simulink model "Block_diagram"  (R2018b)
settings: Solver=VariableStepAuto  StartTime=0.0  StopTime=10  FixedStep=1e-6  RelTol=1e-3
undefined symbols (not defined in the file): sigbuilder_block
libraries: simulink x2
settings Model: Creator=Anmol Kathail  LastModifiedBy=Anmol Kathail

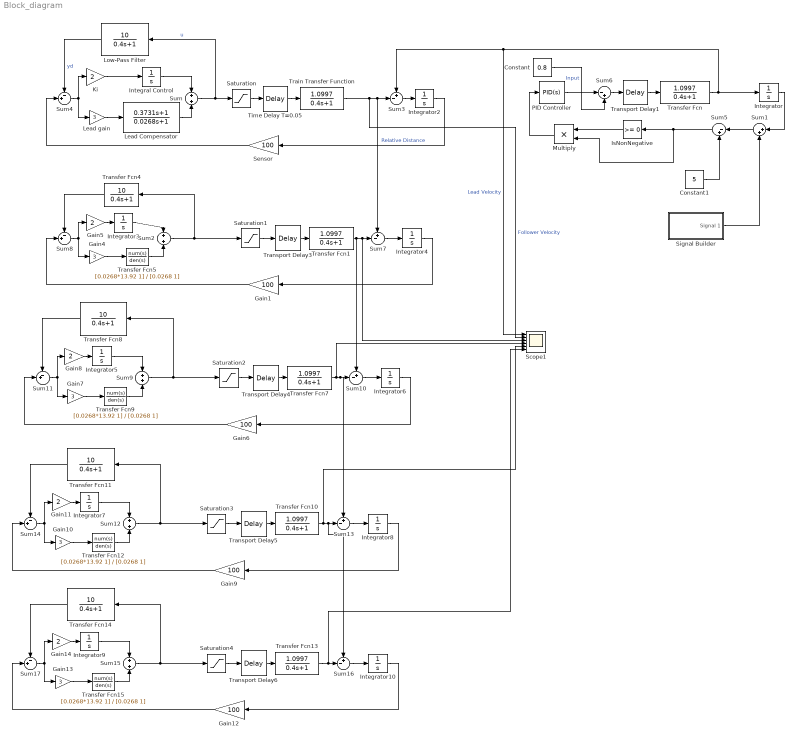
== system Block_diagram ==
  Constant : Constant  Value=0.8
  Constant1 : Constant  Value=5
  Gain{1,6,9,12} (4 alike) : Gain  Gain=100
  Gain{4,7,10,13} (4 alike) : Gain  Gain=3
  Gain{5,8,11,14} (4 alike) : Gain  Gain=2
  Integral Control : Integrator
  Integrator{,2..10} (10 alike) : Integrator
  IsNonNegative : simulink/Logic and Bit Operations/Compare To Zero  relop=>=  OutDataTypeStr=boolean
  Ki : Gain  Gain=2
  Lead Compensator : TransferFcn  Numerator=[0.3731 1]  Denominator=[0.0268 1]
  Lead gain : Gain  Gain=3
  Low-Pass Filter : TransferFcn  Numerator=[10]  Denominator=[0.4 1]
  Multiply : Product
  PID Controller : simulink/Continuous/PID Controller  Controller=PID  Form=Parallel  TimeDomain=Continuous-time  SampleTime=-1  IntegratorMethod=Forward Euler  FilterMethod=Forward Euler  ControllerParametersSource=internal  P=0.1  I=0  D=0  UseFilter=on  N=100  TunerSelectOption=Transfer Function Based (PID Tuner App)  InitialConditionSource=internal  InitialConditionForIntegrator=0  InitialConditionForFilter=0  DifferentiatorICPrevScaledInput=0  ExternalReset=none  TrackingMode=off  Kt=1  LimitOutput=off  UpperSaturationLimit=inf  LowerSaturationLimit=-inf  LinearizeAsGain=on  AntiWindupMode=none  Kb=1  POutMin=[]  POutMax=[]  IOutMin=[]  IOutMax=[]  DOutMin=[]  DOutMax=[]  NOutMin=[]  NOutMax=[]  SumOutMin=[]  SumOutMax=[]  SaturationOutMin=[]  SaturationOutMax=[]  PParamMin=[]  PParamMax=[]  IParamMin=[]  IParamMax=[]  DParamMin=[]  DParamMax=[]  NParamMin=[]  NParamMax=[]  KbParamMin=[]  KbParamMax=[]  KtParamMin=[]  KtParamMax=[]  KbOutMin=[]  KbOutMax=[]  KtOutMin=[]  KtOutMax=[]  IntegratorOutMin=[]  IntegratorOutMax=[]  FilterOutMin=[]  FilterOutMax=[]  SumI1OutMin=[]  SumI1OutMax=[]  SumI2OutMin=[]  SumI2OutMax=[]  SumI3OutMin=[]  SumI3OutMax=[]  SumI4OutMin=[]  SumI4OutMax=[]  SumDOutMin=[]  SumDOutMax=[]  DifferentiatorOutMin=[]  DifferentiatorOutMax=[]  FilterDiffOutCoefMin=[]  FilterDiffOutCoefMax=[]  ReciprocalOutMin=[]  ReciprocalOutMax=[]  SumDenOutMin=[]  SumDenOutMax=[]  SumNumOutMin=[]  SumNumOutMax=[]  DivideOutMin=[]  DivideOutMax=[]  IntegratorContinuousStateAttributes=''  IntegratorStateMustResolveToSignalObject=off  IntegratorRTWStateStorageClass=Auto  FilterContinuousStateAttributes=''  FilterStateMustResolveToSignalObject=off  FilterRTWStateStorageClass=Auto  ParallelPVariant=InternalParameters  IdealPVariant=Disabled  IVariant=InternalParameters  DVariant=InternalParameters  IntegratorVariant=Continuous  SatVariant=Disabled  AWVariant=Passthrough  PCopyVariant=Disabled  TRVariant=Disabled  FdbkBlocksVariant=Forward  IdealPFdbkVariant=Disabled  SatFdbkVariant=Disabled  DerivativeFilterVariant=ContFilter  NVariant=InternalParameters  NCopyVariant=Disabled  FilterICVariant=InternalICsFilter  IntegratorICVariant=InternalICs  ExternalResetVariant=Disabled  TRSumVariant=Passthrough  SumFdbkVariant=Disabled  SumVariant=Sum_PID
  Saturation{,1..4} (5 alike) : Saturate  UpperLimit=1  LowerLimit=0
  Scope1 : Scope  NumInputPorts=6
  Sensor : Gain  Gain=100
  Signal Builder : Subsystem  Tag=STV Subsys  LoadFcn=sigbuilder_block('load',[242.25 90 550.5 359.25 ]);  StartFcn=sigbuilder_block('start');  StopFcn=sigbuilder_block('stop');  ClipboardFcn=sigbuilder_block('clipboard');  mask(Sigbuilder block){tuvar=[0:10]}
      mask help: Simulink:masks:SigbuilderBlock_MD
      mask init:
      | if ~strcmp(get_param(bdroot(gcbh),'SimulationStatus'),'stopped') tuvar = sigbuilder_block('maskInit'); end
      settings: CopyFcn=sigbuilder_block('copy');  DeleteFcn=sigbuilder_block('delete');  ModelCloseFcn=sigbuilder_block('modelClose');  PreSaveFcn=sigbuilder_block('preSave');  PauseFcn=sigbuilder_block('pause');  ContinueFcn=sigbuilder_block('continue');  NameChangeFcn=sigbuilder_block('namechange');  OpenFcn=sigbuilder_block('open',[242.25 90 550.5 359.25 ]);  CloseFcn=sigbuilder_block('close');
      mask Display: plot(0, 0, 100, 100,[2, 2, 32, 32, 2], [68, 8, 8, 68, 68],[32, 2], [38, 38], [32, 19, 2],[53, 60, 44], [32, 17, 17, 2],[16, 16, 31, 31]);txt = getActiveGroup(gcbh);text(2, 100, txt,'verticalAlignment', 'top');
  Sum{,2,9,12,15} (5 alike) : Sum  Inputs=+|+
  Sum1 : Sum  Inputs=|++
  Sum{3,7,10,13,16} (5 alike) : Sum  Inputs=+-|
  Sum{4,8,11,14,17} (5 alike) : Sum  Inputs=-+|
  Sum5 : Sum  Inputs=|-+
  Sum6 : Sum  Inputs=|-+
  Time Delay T=0.05 : TransportDelay  DelayTime=0.05  PadeOrder=3
  Train Transfer Function : TransferFcn  Numerator=[1.0997]  Denominator=[0.4 1]
  Transfer Fcn{,1,7,10,13} (5 alike) : TransferFcn  Numerator=[1.0997]  Denominator=[0.4 1]
  Transfer Fcn{4,8,11,14} (4 alike) : TransferFcn  Numerator=[10]  Denominator=[0.4 1]
  Transfer Fcn{5,9,12,15} (4 alike) : TransferFcn  Numerator=[0.0268*13.92 1]  Denominator=[0.0268 1]
  Transport Delay{1,3..6} (5 alike) : TransportDelay  DelayTime=0.05  PadeOrder=3
  wires:
  IsNonNegative/1 -> Multiply/1
  Low-Pass Filter/1 -> Sum4/1  "yd"
  Sum3/1 -> Integrator2/1
  Constant1/1 -> Sum5/2
  Sum5/1 -> Multiply/2, IsNonNegative/1
  PID Controller/1 -> Sum6/1
  Multiply/1 -> PID Controller/1
  Sum1/1 -> Sum5/1
  Integrator/1 -> Sum1/1
  Sum6/1 -> Transport Delay1/1
  Transport Delay1/1 -> Transfer Fcn/1
  Time Delay T=0.05/1 -> Train Transfer Function/1
  Signal Builder/1(Signal 1) -> Sum1/2
  Saturation/1 -> Time Delay T=0.05/1
  Integrator2/1 -> Sensor/1  "Relative Distance"
  Ki/1 -> Integral Control/1
  Sum4/1 -> Lead gain/1, Ki/1
  Integral Control/1 -> Sum/1
  Sum/1 -> Low-Pass Filter/1, Saturation/1  "u"
  Lead gain/1 -> Lead Compensator/1
  Lead Compensator/1 -> Sum/2
  Transfer Fcn/1 -> Scope1/1, Sum3/1, Integrator/1  "Lead Velocity"
  Sensor/1 -> Sum4/2
  Transfer Fcn1/1 -> Scope1/3, Sum7/2, Sum10/1
  Gain4/1 -> Transfer Fcn5/1
  Transfer Fcn5/1 -> Sum2/2
  Sum8/1 -> Gain4/1, Gain5/1
  Gain5/1 -> Integrator3/1
  Integrator4/1 -> Gain1/1
  Sum7/1 -> Integrator4/1
  Sum2/1 -> Transfer Fcn4/1, Saturation1/1
  Transport Delay3/1 -> Transfer Fcn1/1
  Integrator3/1 -> Sum2/1
  Saturation1/1 -> Transport Delay3/1
  Transfer Fcn4/1 -> Sum8/1
  Gain1/1 -> Sum8/2
  Transfer Fcn8/1 -> Sum11/1
  Saturation2/1 -> Transport Delay4/1
  Gain6/1 -> Sum11/2
  Transport Delay4/1 -> Transfer Fcn7/1
  Integrator5/1 -> Sum9/1
  Sum10/1 -> Integrator6/1
  Integrator6/1 -> Gain6/1
  Transfer Fcn7/1 -> Scope1/4, Sum13/1, Sum10/2
  Gain8/1 -> Integrator5/1
  Transfer Fcn9/1 -> Sum9/2
  Sum11/1 -> Gain7/1, Gain8/1
  Sum9/1 -> Transfer Fcn8/1, Saturation2/1
  Gain7/1 -> Transfer Fcn9/1
  Transfer Fcn11/1 -> Sum14/1
  Saturation3/1 -> Transport Delay5/1
  Gain9/1 -> Sum14/2
  Transport Delay5/1 -> Transfer Fcn10/1
  Integrator7/1 -> Sum12/1
  Sum13/1 -> Integrator8/1
  Integrator8/1 -> Gain9/1
  Transfer Fcn10/1 -> Scope1/5, Sum16/1, Sum13/2
  Gain11/1 -> Integrator7/1
  Transfer Fcn12/1 -> Sum12/2
  Sum14/1 -> Gain10/1, Gain11/1
  Sum12/1 -> Transfer Fcn11/1, Saturation3/1
  Gain10/1 -> Transfer Fcn12/1
  Transfer Fcn14/1 -> Sum17/1
  Saturation4/1 -> Transport Delay6/1
  Gain12/1 -> Sum17/2
  Transport Delay6/1 -> Transfer Fcn13/1
  Integrator9/1 -> Sum15/1
  Sum16/1 -> Integrator10/1
  Integrator10/1 -> Gain12/1
  Gain14/1 -> Integrator9/1
  Transfer Fcn15/1 -> Sum15/2
  Sum17/1 -> Gain13/1, Gain14/1
  Sum15/1 -> Transfer Fcn14/1, Saturation4/1
  Gain13/1 -> Transfer Fcn15/1
  Transfer Fcn13/1 -> Scope1/6, Sum16/2
  Train Transfer Function/1 -> Scope1/2, Sum7/1, Sum3/2  "Follower Velocity"
  Constant/1 -> Sum6/2  "Input"

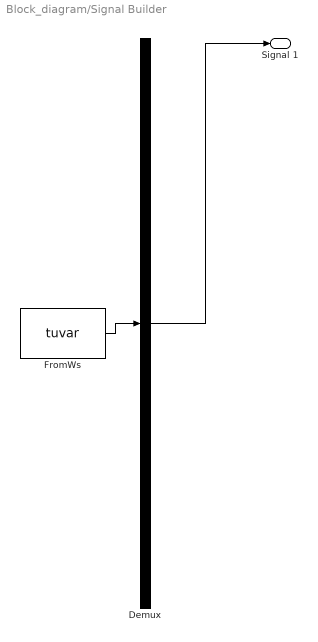
== system Block_diagram/Signal Builder ==
  Demux : Demux  Tag=STV Demux  Outputs=1
  FromWs : FromWorkspace  Tag=STV FromWs  VariableName=tuvar  SampleTime=0
      SigBuilderData=|
      | common.afterFinalStr = 'Extrapolate'
      | common.sampleTime = 0
      | dataSet.timeRange = [0 10]
      | dataSet.name = 'Group 1'
      | sbobj.Groups.Name = 'Group 1'
      | sbobj.Groups.Signals.Name = 'Signal 1'
      | sbobj.Groups.Signals.XData = [0 0.0625 0.125 0.1875 0.25 0.3125 0.375 0.4375 0.5 0.5625 0.625 0.6875 0.75 0.8125 0.875 0.9375 1 1.0625 1.125 1.1875 1.25 1.3125 1.375 1.4375 1.5 1.5625 1.625 1.6875 1.75 1.8125 1.875 1.9375 2 2.0625 2.125 2.1875 2.25 2.3125 2.375 2.4375 2.5 2.5625 2.625 2.6875 2.75 2.8125 2.875 2.9375 3 3.0625 3.125 3.1875 3.25 3.3125 3.375 3.4375 3.5 3.5625 3.625 3.6875 3.75 3.8125 3.875 3.9375 4 4.0625 4.125 4.1875 4.25 4.3125 4.375 4.4375 4.5 4.5625 4.625 4.6875 4.75 4.8125 4.875 4.9375 5 5.0625 5.125 5.1875 5.25 5.3125 5.375 5.4375 5.5 5.5625 5.625 5.6875 5.75 5.8125 5.875 5.9375 6 6.0625 6.125 6.1875 6.25 6.3125 6.375 6.4375 6.5 6.5625 6.625 6.6875 6.75 6.8125 6.875 6.9375 7 7.0625 7.125 7.1875 7.25 7.3125 7.375 7.4375 7.5 7.5625 7.625 7.6875 7.75 7.8125 7.875 7.9375 8 8.0625 8.125 8.1875 8.25 8.3125 8.375 8.4375 8.5 8.5625 8.625 8.6875 8.75 8.8125 8.875 8.9375 9 9.0625 9.125 9.1875 9.25 9.3125 9.375 9.4375 9.5 9.5625 9.625 9.6875 9.75 9.8125 9.875 9.9375 10]
      | sbobj.Groups.Signals.YData = [5 6.41421356237 7 6.41421356237 5 3.58578643763 3 3.58578643763 5 6.41421356237 7 6.41421356237 5 3.58578643763 3 3.58578643763 5 6.41421356237 7 6.41421356237 5 3.58578643763 3 3.58578643763 5 6.41421356237 7 6.41421356237 5 3.58578643763 3 3.58578643763 5 6.41421356237 7 6.41421356237 5 3.58578643763 3 3.58578643763 5 6.41421356237 7 6.41421356237 5 3.58578643763 3 3.58578643763 5 6.41421356237 7 6.41421356237 5 3.58578643763 3 3.58578643763 5 6.41421356237 7 6.41421356237 5 3.58578643763 3 3.58578643763 5 6.41421356237 7 6.41421356237 5 3.58578643763 3 3.58578643763 5 6.41421356237 7 6.41421356237 5 3.58578643763 3 3.58578643763 5 6.41421356237 7 6.41421356237 5 3.58578643763 3 3.58578643763 5 6.41421356237 7 6.41421356237 5 3.58578643763 3 3.58578643763 5 6.41421356237 7 6.41421356237 5 3.58578643763 3 3.58578643763 5 6.41421356237 7 6.41421356237 5 3.58578643763 3 3.58578643763 5 6.41421356237 7 6.41421356237 5 3.58578643763 3 3.58578643763 5 6.41421356237 7 6.41421356237 5 3.58578643763 3 3.58578643763 5 6.41421356237 7 6.41421356237 5 3.58578643763 3 3.58578643763 5 6.41421356237 7 6.41421356237 5 3.58578643763 3 3.58578643763 5 6.41421356237 7 6.41421356237 5 3.58578643763 3 3.58578643763 5 6.41421356237 7 6.41421356237 5 3.58578643763 3 3.58578643763 5]
  Signal 1 : Outport  Tag=STV Outport
  wires:
  Demux/1 -> Signal 1/1
  FromWs/1 -> Demux/1
